simulink model "simu_discreta_2018"  (R2018b)
settings: Solver=VariableStepAuto  StartTime=0.0  StopTime=10.0  RelTol=1e-3
undefined symbols (not defined in the file): Kd, sysd
settings Model: Creator=valac  LastModifiedBy=valac
settings DataIOCC: ReturnWorkspaceOutputs=on

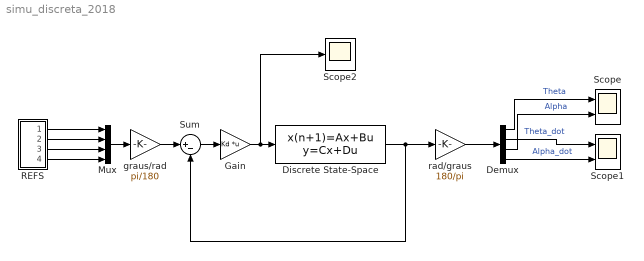
== system simu_discreta_2018 ==
  Demux : Demux
  Discrete State-Space : DiscreteStateSpace  A=sysd.A  B=sysd.B  C=eye(4)  D=zeros(4,1)  InitialCondition=[0 0 10*pi/180 0]  SampleTime=1/10
  Gain : Gain  Gain=Kd  Multiplication=Matrix(K*u)
  Mux : Mux
  REFS : Subsystem
  Scope : Scope  NumInputPorts=2
  Scope1 : Scope  NumInputPorts=2
  Scope2 : Scope
  Sum : Sum  Inputs=|+-
  graus/rad : Gain  Gain=pi/180
  rad/graus : Gain  Gain=180/pi
  wires:
  Sum/1 -> Gain/1
  Demux/1 -> Scope/1  "Theta"
  Demux/2 -> Scope1/1  "Theta_dot"
  Demux/3 -> Scope/2  "Alpha"
  Demux/4 -> Scope1/2  "Alpha_dot"
  Gain/1 -> Scope2/1, Discrete State-Space/1
  Mux/1 -> graus/rad/1
  rad/graus/1 -> Demux/1
  graus/rad/1 -> Sum/1
  REFS/1(Out1) -> Mux/1
  REFS/2(Out2) -> Mux/2
  REFS/3(Out3) -> Mux/3
  REFS/4(Out4) -> Mux/4
  Discrete State-Space/1 -> Sum/2, rad/graus/1

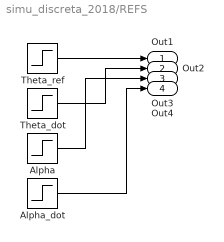
== system simu_discreta_2018/REFS ==
  Alpha : Step  Time=0.5  After=0  SampleTime=0
  Alpha_dot : Step  After=0  SampleTime=0
  Theta_dot : Step  After=0  SampleTime=0
  Theta_ref : Step  After=0  SampleTime=0
  Out1 : Outport
  Out2 : Outport  Port=2
  Out3 : Outport  Port=3
  Out4 : Outport  Port=4
  wires:
  Alpha/1 -> Out3/1
  Theta_ref/1 -> Out1/1
  Alpha_dot/1 -> Out4/1
  Theta_dot/1 -> Out2/1
